simulink model "Function22"  (Simulink 8.8)
settings: Solver=VariableStepAuto  StartTime=0.0  StopTime=10.0  RelTol=1e-3
undefined symbols (not defined in the file): F11CONST, F21CONST, F22CONST, MFMdl2CONST
libraries: simulink x2
settings Model: Creator=viett  LastModifiedBy=viett
settings DataIOCC: LimitDataPoints=off  SaveFormat=Dataset  SignalLoggingSaveFormat=Dataset
settings OptimizationCC: LifeSpan=auto
settings DebuggingCC: UnderspecifiedInitializationDetection=Simplified  MergeDetectMultiDrivingBlocksExec=error  FcnCallInpInsideContextMsg=error  StateNameClashWarn=none  SFUnexpectedBacktrackingDiag=error  SFNoUnconditionalDefaultTransitionDiag=error  SFExecutionAtInitializationDiag=warning
settings HardwareCC: ProdBitPerPointer=64  ProdBitPerSizeT=64  ProdBitPerPtrDiffT=64  ProdLargestAtomicFloat=Float  ProdIntDivRoundTo=Zero  ProdEndianess=LittleEndian  ProdWordSize=64  ProdHWDeviceType=Intel->x86-64 (Windows64)
settings ModelReferenceCC: PropagateSignalLabelsOutOfModel=on
settings GRTTargetCC: TargetLangStandard=C99 (ISO)  GeneratePreprocessorConditionals=Use local settings  CombineOutputUpdateFcns=on  GRTInterface=off
settings ConfigComp: CovMetricSettings=dwe  CovHtmlReporting=off  CovSaveCumulativeToWorkspaceVar=off  CovSaveSingleToWorkspaceVar=off  CovExternalEMLEnable=on

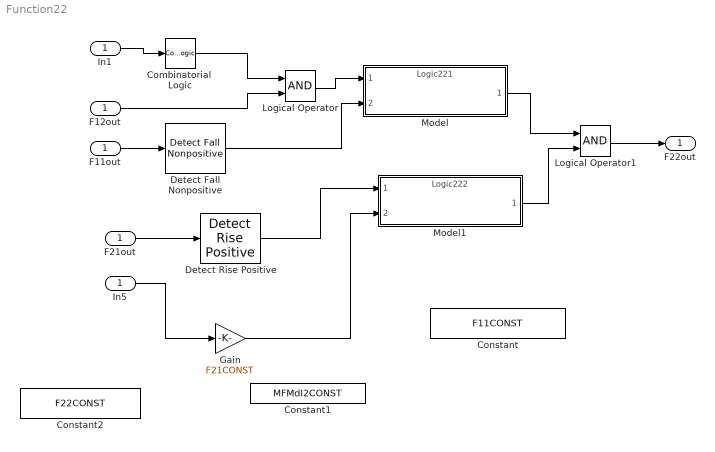
== system Function22 ==
  In1 : Inport
  Combinatorial  Logic : CombinatorialLogic
  Constant : Constant  Value=F11CONST
  Constant1 : Constant  Value=MFMdl2CONST
  Constant2 : Constant  Value=F22CONST
  Detect Fall Nonpositive : simulink/Logic and Bit Operations/Detect Fall Nonpositive  vinit=0  OutDataTypeStr=boolean
  Detect Rise Positive : simulink/Logic and Bit Operations/Detect Rise Positive  vinit=0  OutDataTypeStr=boolean
  F11out : InportShadow
  F12out : InportShadow
  F21out : InportShadow
  Gain : Gain  Gain=F21CONST
  In5 : InportShadow
  Logical Operator : Logic  AllPortsSameDT=off  OutDataTypeStr=boolean
  Logical Operator1 : Logic  AllPortsSameDT=off  OutDataTypeStr=boolean
  Model : ModelReference  ModelNameDialog=Logic221.slx  SimulationMode=Normal  ModelReferenceVersion=1.2
  Model1 : ModelReference  ModelNameDialog=Logic222.slx  SimulationMode=Normal  ModelReferenceVersion=1.2
  F22out : Outport
  wires:
  Logical Operator/1 -> Model/1
  Detect Fall Nonpositive/1 -> Model/2
  Combinatorial  Logic/1 -> Logical Operator/1
  In1/1 -> Combinatorial  Logic/1
  F12out/1 -> Logical Operator/2
  F11out/1 -> Detect Fall Nonpositive/1
  Model/1 -> Logical Operator1/1
  Logical Operator1/1 -> F22out/1
  Model1/1 -> Logical Operator1/2
  Detect Rise Positive/1 -> Model1/1
  F21out/1 -> Detect Rise Positive/1
  Gain/1 -> Model1/2
  In5/1 -> Gain/1
